simulink model "FinalLab3"  (R2018a)
settings: Solver=VariableStepAuto  StartTime=0.0  StopTime=.2  RelTol=1e-3
undefined symbols (not defined in the file or in its folder): DiscIntNeverNeededParam
libraries: dsparch4 x1, commsynccomp2 x1, dspsrcs4 x1
settings Model: Creator=salman  LastModifiedBy=Salman Prottoy

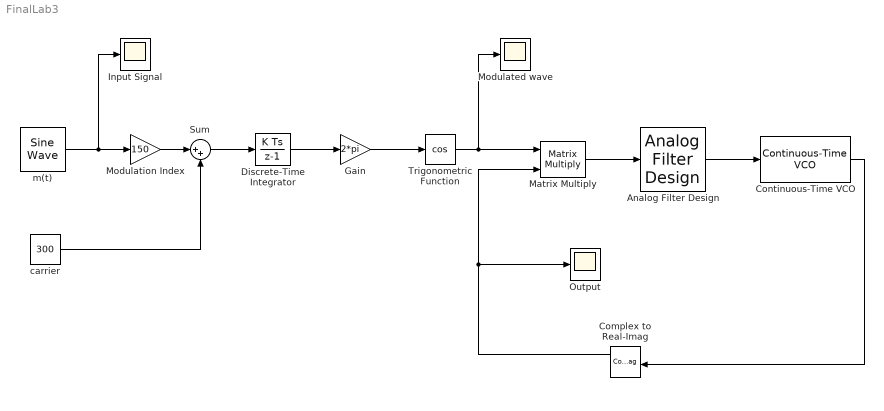
== system FinalLab3 ==
  "Analog Filter Design " : dsparch4/Analog Filter Design  method=Butterworth  filttype=Lowpass  N=10  Wlo=2*pi*10  Whi=80  Rp=2  Rs=40
  "Complex to Real-Imag " : ComplexToRealImag
  "Continuous-Time VCO " : commsynccomp2/Continuous-Time VCO  Ac=1  Fc=10  Kc=50  Ph=0
      settings: SourceProductName=Communications System Toolbox  SourceProductBaseCode=CM
  "Discrete-Time Integrator " : DiscreteIntegrator  SampleTime=1/98000  ICPrevOutput=DiscIntNeverNeededParam  ICPrevScaledInput=DiscIntNeverNeededParam
  "Gain " : Gain  Gain=2*pi
  Input Signal : Scope
  "Matrix Multiply " : Product  Multiplication=Matrix(*)
  Modulated wave : Scope
  Modulation Index : Gain  Gain=150
  Output : Scope
  Sum : Sum  Inputs=|++
  "Trigonometric Function " : Trigonometry  Operator=cos
  carrier : Constant  Value=300
  m(t) : dspsrcs4/Sine Wave  Amplitude=1  Frequency=10  Phase=90  SampleMode=Discrete  OutComplex=Real  CompMethod=Trigonometric fcn  TableSize=Speed  SampleTime=1/98000  SamplesPerFrame=1  ResetState=Restart at time zero  OutputFrames=off  dataType=double  wordLen=16  udDataType=sfix(16)  fracBitsMode=Best precision  numFracBits=15  OutDataTypeStr=double  LastOutDataTypeStr=double
  wires:
  carrier/1 -> Sum/2
  Modulation Index/1 -> Sum/1
  m(t)/1 -> Input Signal/1, Modulation Index/1
  "Trigonometric Function "/1 -> Modulated wave/1, "Matrix Multiply "/1
  "Gain "/1 -> "Trigonometric Function "/1
  Sum/1 -> "Discrete-Time Integrator "/1
  "Discrete-Time Integrator "/1 -> "Gain "/1
  "Analog Filter Design "/1 -> "Continuous-Time VCO "/1
  "Matrix Multiply "/1 -> "Analog Filter Design "/1
  "Continuous-Time VCO "/1 -> "Complex to Real-Imag "/1
  "Complex to Real-Imag "/1 -> "Matrix Multiply "/2, Output/1
